simulink model "simulink_discrete_2_R2021a"  (R2021a)
settings: Solver=ode23  StartTime=0.0  StopTime=0.7  FixedStep=T1  MaxStep=1E-5  RelTol=1e-3  EnableMultiTasking=on
undefined symbols (not defined in the file): T1, T2
libraries: cstblocks x6
settings Model: Creator=Koldo  LastModifiedBy=Koldo
settings SolverCC: ShapePreserveControl=EnableAll  ZeroCrossAlgorithm=Adaptive  AlgebraicLoopSolver=TrustRegion  PositivePriorityOrder=on  AutoInsertRateTranBlk=on  InsertRTBMode=Never (minimum delay)
settings DataIOCC: LimitDataPoints=on  SaveFormat=Array  SignalLoggingSaveFormat=ModelDataLogs  ReturnWorkspaceOutputs=off
settings OptimizationCC: ExpressionDepthLimit=2147483647  LifeSpan=inf
settings DebuggingCC: UnderspecifiedInitializationDetection=Classic  MergeDetectMultiDrivingBlocksExec=none  IgnoredZcDiagnostic=none  SolverPrmCheckMsg=warning  FcnCallInpInsideContextMsg=warning  StateNameClashWarn=warning  SFUnexpectedBacktrackingDiag=warning  SFNoUnconditionalDefaultTransitionDiag=warning  SFExecutionAtInitializationDiag=none  SFMachineParentedDataDiag=warning  ArithmeticOperatorsInVariantConditions=warning
settings HardwareCC: ProdBitPerPointer=32  ProdBitPerSizeT=32  ProdBitPerPtrDiffT=32  ProdLargestAtomicFloat=None  ProdIntDivRoundTo=Undefined  ProdEndianess=Unspecified  ProdWordSize=32  ProdHWDeviceType=32-bit Generic
settings ModelReferenceCC: PropagateSignalLabelsOutOfModel=off
settings SFSimCC: SimUseLocalCustomCode=off  CustomCodeUndefinedFunction=UseInterfaceOnly
settings RTWCC: RTWUseLocalCustomCode=off
settings CodeAppCC: StateflowObjectComments=on
settings GRTTargetCC: TargetLangStandard=C89/C90 (ANSI)  CombineOutputUpdateFcns=off  GRTInterface=on
settings ConfigComp: CovMetricSettings=dw  CovSaveCumulativeToWorkspaceVar=on  CovSaveSingleToWorkspaceVar=on  CovExternalEMLEnable=off

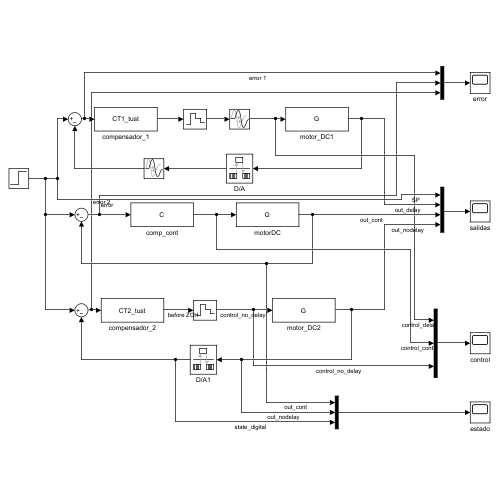
[thumbnail: Simulink's stored preview of the top-level diagram]
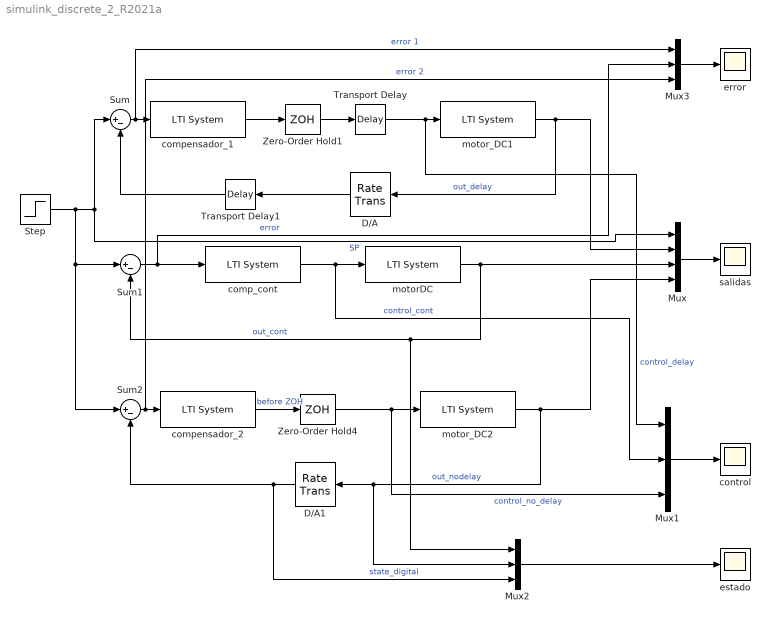
== system simulink_discrete_2_R2021a ==
  D/A : RateTransition  Priority=0  Integrity=off  Deterministic=off  OutPortSampleTime=T1
  D/A1 : RateTransition  Integrity=off  Deterministic=off  OutPortSampleTime=T2
  Mux : Mux
  Mux1 : Mux  Inputs=3
  Mux2 : Mux  Inputs=3
  Mux3 : Mux  Inputs=3
  Step : Step  Time=0.1  After=pi/2  SampleTime=0
  Sum : Sum  Inputs=|+-
  Sum1 : Sum  Inputs=|+-
  Sum2 : Sum  Inputs=|+-
  Transport Delay : TransportDelay  DelayTime=1.2*T1
  Transport Delay1 : TransportDelay  DelayTime=0
  Zero-Order Hold1 : ZeroOrderHold  SampleTime=T1
  Zero-Order Hold4 : ZeroOrderHold  SampleTime=T2
  comp_cont : cstblocks/LTI System  sys=C  IC=[]
  compensador_1 : cstblocks/LTI System  Priority=1  sys=CT1_tust  IC=[]
  compensador_2 : cstblocks/LTI System  Priority=1  sys=CT2_tust  IC=[]
  control : Scope
  error : Scope
  estado : Scope
  motorDC : cstblocks/LTI System  sys=G  IC=[]
  motor_DC1 : cstblocks/LTI System  sys=G  IC=[]
  motor_DC2 : cstblocks/LTI System  sys=G  IC=[]
  salidas : Scope
  wires:
  Sum/1 -> Mux3/1, compensador_1/1  "error 1"
  compensador_1/1 -> Zero-Order Hold1/1
  Sum1/1 -> Mux3/2, comp_cont/1  "error"
  motorDC/1 -> Mux/3, Mux2/1, Sum1/2  "out_cont"
  comp_cont/1 -> motorDC/1, Mux1/2  "control_cont"
  Mux/1 -> salidas/1
  Step/1 -> Sum1/1, Sum2/1, Sum/1, Mux/1  "SP"
  Sum2/1 -> Mux3/3, compensador_2/1  "error 2"
  Zero-Order Hold4/1 -> motor_DC2/1, Mux1/3  "control_no_delay"
  Mux1/1 -> control/1
  motor_DC1/1 -> D/A/1, Mux/2  "out_delay"
  compensador_2/1 -> Zero-Order Hold4/1  "before ZOH"
  Zero-Order Hold1/1 -> Transport Delay/1
  Transport Delay/1 -> motor_DC1/1, Mux1/1  "control_delay"
  Transport Delay1/1 -> Sum/2
  D/A/1 -> Transport Delay1/1
  motor_DC2/1 -> Mux2/2, D/A1/1, Mux/4  "out_nodelay"
  Mux2/1 -> estado/1
  D/A1/1 -> Sum2/2, Mux2/3  "state_digital"
  Mux3/1 -> error/1
